simulink model "test_simmechanics_handling"  (Simulink 6.4)
settings: Solver=ode45  StartTime=0.0  StopTime=10  RelTol=1e-4  AbsTol=1e-4
InitFcn:
  | hFA = 0.2908;
  | hRA = 0.2909;
StopFcn:
  | subplot(3,1,1)
  | plot(time,velacc(:,8))
  | ylabel('lateral acceleration [m/s2]')
  | 
  | subplot(3,1,2)
  | plot(time,velacc(:,6))
  | ylabel('yaw velocity [deg/s]')
  | 
  | subplot(3,1,3)
  | plot(time,varinf1(:,3),time,varinf2(:,3),time,varinf3(:,3),time,varinf4(:,3))
  | xlabel('time [s]')
  | ylabel('vertical tyre force Fz [N]')
libraries: mblibv1 x31, Delft_Tyre_sm1glib x12
settings Model: Creator=luijtenmfj  LastModifiedBy=hofstadrhmtvd
settings DataIOCC: LimitDataPoints=off  SaveOutput=off  SignalLoggingName=sigsOut  OutputOption=SpecifiedOutputTimes  OutputTimes=[0:0.01:10]
settings DebuggingCC: SolverPrmCheckMsg=none  StrictBusMsg=ErrorLevel1
settings HardwareCC: TargetEndianess=LittleEndian  TargetHWDeviceType=MATLAB Host  ProdEqTarget=off
settings RTWCC: SystemTargetFile=rsim.tlc  TemplateMakefile=rsim_default_tmf  Description=Rapid Simulation Target  ProcessScript=rsim_make_rtw_hook
settings RSimTargetCC: TargetFcnLib=ansi_tfl_tmw.mat  GenFloatMathFcnCalls=ANSI_C  IsPILTarget=off  IncludeERTFirstTime=on
settings CustomProperty: DataType=string  Value=ANSI_C
settings SimMechanicsCC: VisDuringSimulation=on

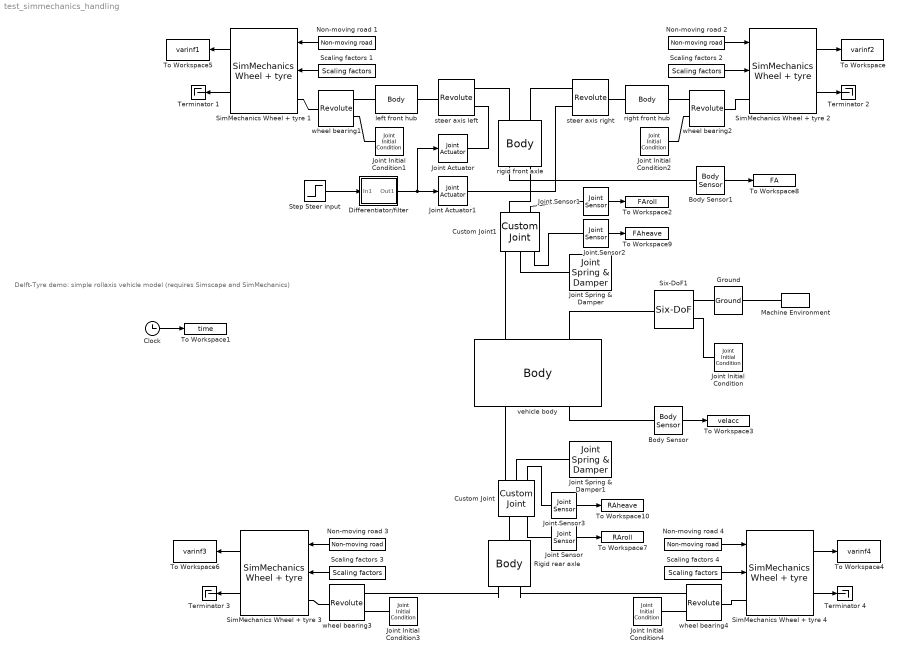
== system test_simmechanics_handling ==
  note: Delft-Tyre demo: simple rollaxis vehicle model
      | (requires Simscape and SimMechanics)
  Body Sensor : mblibv1/Sensors &  Actuators/Body Sensor  DialogController=MECH.DynMechDlgSource  SystemSampleTime=-1  PhysicalDomain=Mechanical  PortType=blob  Muxed=on  Pose=off  Angle=on  AngleUnits=deg  ArcVelocity=on  ArcVelocityUnits=deg/s  ArcAcceleration=off  ArcAccelerationUnits=deg/s^2  CoordPosition=off  CoordPositionUnits=m  Velocity=on  VelocityUnits=m/s  Acceleration=on  AccelerationUnits=m/s^2  Quaternion=on  QuaternionDT=off  QuaternionDDT=off  QuaternionUnits=off  OutputVector=[ 3 3 3 ]  ActiveIO=on  Width=9  DialogClass=MechanicalSensorBlock  ReferenceFrame=Local (Body CS)
  Body Sensor1 : mblibv1/Sensors &  Actuators/Body Sensor  DialogController=MECH.DynMechDlgSource  SystemSampleTime=-1  PhysicalDomain=Mechanical  PortType=blob  Muxed=on  Pose=off  Angle=on  AngleUnits=deg  ArcVelocity=off  ArcVelocityUnits=deg/s  ArcAcceleration=off  ArcAccelerationUnits=deg/s^2  CoordPosition=on  CoordPositionUnits=m  Velocity=off  VelocityUnits=m/s  Acceleration=off  AccelerationUnits=m/s^2  Quaternion=on  QuaternionDT=off  QuaternionDDT=off  QuaternionUnits=off  OutputVector=[ 3 ]  ActiveIO=on  Width=3  DialogClass=MechanicalSensorBlock  ReferenceFrame=Absolute (World)
  Clock : Clock
      settings: Decimation=10
  Custom Joint : mblibv1/Joints/Custom Joint  Orientation=down  DialogController=MECH.DynMechDlgSource  PhysicalDomain=mechanical  SubClassName=custom_joint  LeftPortType=blob  RightPortType=blob  LConnTagsString=__newl0|SA1|SA2  RConnTagsString=__newr0|SA1  NumSAPorts=3  CutJoint=off  MarkAsCut=off  Primitives=prismatic_revolute  PrimitiveProps=P1$WORLD$[0 0 1]$prismatic#R1$WORLD$[1 0 0]$revolute  DialogClass=JointBlock
  Custom Joint1 : mblibv1/Joints/Custom Joint  Orientation=up  DialogController=MECH.DynMechDlgSource  PhysicalDomain=mechanical  SubClassName=custom_joint  LeftPortType=blob  RightPortType=blob  LConnTagsString=__newl0|SA1|SA2  RConnTagsString=__newr0|SA1  NumSAPorts=3  CutJoint=off  MarkAsCut=off  Primitives=prismatic_revolute  PrimitiveProps=P1$WORLD$[0 0 1]$prismatic#R1$WORLD$[1 0 0]$revolute  DialogClass=JointBlock
  Differentiator/filter : Subsystem  mask{ts=0.05}
      mask prompts: ts "response_time"
      mask init:
      | c=(3*pi/ts)^2;
  Ground : mblibv1/Bodies/Ground  Orientation=left  DialogController=MECH.DynMechDlgSource  SystemSampleTime=-1  LeftPortType=env  RightPortType=workingframe  PhysicalDomain=Mechanical  DialogClass=GroundBlock  CoordPosition=[0 0 0]  CoordPositionUnits=m  StateVectorMgrId=-1  MachineId=[0 0]  ShowEnvPort=on
  Joint Actuator : mblibv1/Sensors &  Actuators/Joint Actuator  DialogController=MECH.DynMechDlgSource  SystemSampleTime=-1  PhysicalDomain=Mechanical  PortType=blob  ActuationStyle=Motion  AngleUnits=rad  ArcVelocityUnits=rad/s  ArcAccelerationUnits=rad/s^2  CoordPositionUnits=m  VelocityUnits=m/s  AccelerationUnits=m/s^2  ForceUnits=N  TorqueUnits=N-m  ActiveIO=on  Width=3  DialogClass=MechanicalActuatorBlock  Primitive=R1  ReferenceFrame=Absolute (INERTIAL)
  Joint Actuator1 : mblibv1/Sensors &  Actuators/Joint Actuator  DialogController=MECH.DynMechDlgSource  SystemSampleTime=-1  PhysicalDomain=Mechanical  PortType=blob  ActuationStyle=Motion  AngleUnits=rad  ArcVelocityUnits=rad/s  ArcAccelerationUnits=rad/s^2  CoordPositionUnits=m  VelocityUnits=m/s  AccelerationUnits=m/s^2  ForceUnits=N  TorqueUnits=N-m  ActiveIO=on  Width=3  DialogClass=MechanicalActuatorBlock  Primitive=R1  ReferenceFrame=Absolute (INERTIAL)
  Joint Initial Condition : mblibv1/Sensors &  Actuators/Joint Initial Condition  Orientation=left  DialogController=MECH.DynMechDlgSource  SystemSampleTime=-1  PhysicalDomain=Mechanical  DialogClass=InitialConditionBlock  InitialConditions=P1$true$0$m$rad$20$m/s$rad/s#P2$false$0$m$rad$0$m/s$rad/s#P3$false$-0.15$m$rad$0$m/s$rad/s#R1$false$0$m$rad$70$m/s$rad/s#R2$false$0$m$rad$0$m/s$rad/s#R3$false$0$m$rad$0$m/s$rad/s#S$false$0$m$rad$0$m/s$rad/s
  Joint Initial Condition1 : mblibv1/Sensors &  Actuators/Joint Initial Condition  Orientation=left  DialogController=MECH.DynMechDlgSource  SystemSampleTime=-1  PhysicalDomain=Mechanical  DialogClass=InitialConditionBlock  InitialConditions=P1$false$0$m$rad$20$m/s$rad/s#P2$false$0$m$rad$0$m/s$rad/s#P3$false$-0.15$m$rad$0$m/s$rad/s#R1$true$0$m$rad$66$m/s$rad/s#R2$false$0$m$rad$0$m/s$rad/s#R3$false$0$m$rad$0$m/s$rad/s#S$false$0$m$rad$0$m/s$rad/s
  Joint Initial Condition2 : mblibv1/Sensors &  Actuators/Joint Initial Condition  DialogController=MECH.DynMechDlgSource  SystemSampleTime=-1  PhysicalDomain=Mechanical  DialogClass=InitialConditionBlock  InitialConditions=P1$false$0$m$rad$20$m/s$rad/s#P2$false$0$m$rad$0$m/s$rad/s#P3$false$-0.15$m$rad$0$m/s$rad/s#R1$true$0$m$rad$66$m/s$rad/s#R2$false$0$m$rad$0$m/s$rad/s#R3$false$0$m$rad$0$m/s$rad/s#S$false$0$m$rad$0$m/s$rad/s
  Joint Initial Condition3 : mblibv1/Sensors &  Actuators/Joint Initial Condition  Orientation=left  DialogController=MECH.DynMechDlgSource  SystemSampleTime=-1  PhysicalDomain=Mechanical  DialogClass=InitialConditionBlock  InitialConditions=P1$false$0$m$rad$20$m/s$rad/s#P2$false$0$m$rad$0$m/s$rad/s#P3$false$-0.15$m$rad$0$m/s$rad/s#R1$true$0$m$rad$66$m/s$rad/s#R2$false$0$m$rad$0$m/s$rad/s#R3$false$0$m$rad$0$m/s$rad/s#S$false$0$m$rad$0$m/s$rad/s
  Joint Initial Condition4 : mblibv1/Sensors &  Actuators/Joint Initial Condition  DialogController=MECH.DynMechDlgSource  SystemSampleTime=-1  PhysicalDomain=Mechanical  DialogClass=InitialConditionBlock  InitialConditions=P1$false$0$m$rad$20$m/s$rad/s#P2$false$0$m$rad$0$m/s$rad/s#P3$false$-0.15$m$rad$0$m/s$rad/s#R1$true$0$m$rad$66$m/s$rad/s#R2$false$0$m$rad$0$m/s$rad/s#R3$false$0$m$rad$0$m/s$rad/s#S$false$0$m$rad$0$m/s$rad/s
  Joint Sensor : mblibv1/Sensors &  Actuators/Joint Sensor  DialogController=MECH.DynMechDlgSource  SystemSampleTime=-1  PhysicalDomain=Mechanical  PortType=blob  Muxed=on  Pose=off  Angle=on  AngleUnits=deg  ArcVelocity=on  ArcVelocityUnits=rad/s  ArcAcceleration=off  ArcAccelerationUnits=deg/s^2  CoordPosition=on  CoordPositionUnits=m  Velocity=off  VelocityUnits=m/s  Acceleration=off  AccelerationUnits=m/s^2  Quaternion=on  QuaternionDT=off  QuaternionDDT=off  QuaternionUnits=off  OutputVector=[ 1 1 3 ]  ActiveIO=on  Width=5  DialogClass=MechanicalSensorBlock  Primitive=R1  Force=off  ForceUnits=N  Torque=off  TorqueUnits=N-m  ReferenceFrame=Absolute (INERTIAL)  ReactionSensedSide=Base  ReactionReferenceFrame=Absolute (World)  ReactionForce=on  ReactionForceUnits=N  ReactionMoment=off  ReactionMomentUnits=N-m
  Joint Sensor1 : mblibv1/Sensors &  Actuators/Joint Sensor  DialogController=MECH.DynMechDlgSource  SystemSampleTime=-1  PhysicalDomain=Mechanical  PortType=blob  Muxed=on  Pose=off  Angle=on  AngleUnits=deg  ArcVelocity=on  ArcVelocityUnits=rad/s  ArcAcceleration=off  ArcAccelerationUnits=deg/s^2  CoordPosition=on  CoordPositionUnits=m  Velocity=off  VelocityUnits=m/s  Acceleration=off  AccelerationUnits=m/s^2  Quaternion=on  QuaternionDT=off  QuaternionDDT=off  QuaternionUnits=off  OutputVector=[ 1 1 3 ]  ActiveIO=on  Width=5  DialogClass=MechanicalSensorBlock  Primitive=R1  Force=off  ForceUnits=N  Torque=off  TorqueUnits=N-m  ReferenceFrame=Absolute (INERTIAL)  ReactionSensedSide=Base  ReactionReferenceFrame=Absolute (World)  ReactionForce=on  ReactionForceUnits=N  ReactionMoment=off  ReactionMomentUnits=N-m
  Joint Sensor2 : mblibv1/Sensors &  Actuators/Joint Sensor  DialogController=MECH.DynMechDlgSource  SystemSampleTime=-1  PhysicalDomain=Mechanical  PortType=blob  Muxed=on  Pose=off  Angle=on  AngleUnits=deg  ArcVelocity=on  ArcVelocityUnits=deg/s  ArcAcceleration=off  ArcAccelerationUnits=deg/s^2  CoordPosition=on  CoordPositionUnits=m  Velocity=on  VelocityUnits=m/s  Acceleration=off  AccelerationUnits=m/s^2  Quaternion=on  QuaternionDT=off  QuaternionDDT=off  QuaternionUnits=off  OutputVector=[ 1 1 3 ]  ActiveIO=on  Width=5  DialogClass=MechanicalSensorBlock  Primitive=P1  Force=off  ForceUnits=N  Torque=off  TorqueUnits=N-m  ReferenceFrame=Absolute (INERTIAL)  ReactionSensedSide=Base  ReactionReferenceFrame=Absolute (World)  ReactionForce=on  ReactionForceUnits=N  ReactionMoment=off  ReactionMomentUnits=N-m
  Joint Sensor3 : mblibv1/Sensors &  Actuators/Joint Sensor  DialogController=MECH.DynMechDlgSource  SystemSampleTime=-1  PhysicalDomain=Mechanical  PortType=blob  Muxed=on  Pose=off  Angle=on  AngleUnits=deg  ArcVelocity=on  ArcVelocityUnits=deg/s  ArcAcceleration=off  ArcAccelerationUnits=deg/s^2  CoordPosition=on  CoordPositionUnits=m  Velocity=on  VelocityUnits=m/s  Acceleration=off  AccelerationUnits=m/s^2  Quaternion=on  QuaternionDT=off  QuaternionDDT=off  QuaternionUnits=off  OutputVector=[ 1 1 3 ]  ActiveIO=on  Width=5  DialogClass=MechanicalSensorBlock  Primitive=P1  Force=off  ForceUnits=N  Torque=off  TorqueUnits=N-m  ReferenceFrame=Absolute (INERTIAL)  ReactionSensedSide=Base  ReactionReferenceFrame=Absolute (World)  ReactionForce=on  ReactionForceUnits=N  ReactionMoment=off  ReactionMomentUnits=N-m
  Joint Spring & Damper : mblibv1/Force  Elements/Joint Spring & Damper  DialogController=MECH.DynMechDlgSource  SystemSampleTime=-1  DialogClass=JointSpringDamper  JFEParameters=P1$true$40000$3500$-.20$m$m/s$N$rad$rad/s$N-m#P2$false$0$0$0$m$m/s$N$rad$rad/s$N-m#P3$false$0$0$0$m$m/s$N$rad$rad/s$N-m#R1$true$66000$2050$0$m$m/s$N$rad$rad/s$N-m#R2$false$0$0$0$m$m/s$N$rad$rad/s$N-m#R3$false$0$0$0$m$m/s$N$rad$rad/s$N-m#S$false$0$0$0$m$m/s$N$rad$rad/s$N-m
  Joint Spring & Damper1 : mblibv1/Force  Elements/Joint Spring & Damper  DialogController=MECH.DynMechDlgSource  SystemSampleTime=-1  DialogClass=JointSpringDamper  JFEParameters=P1$true$50000$3500$-0.16$m$m/s$N$rad$rad/s$N-m#P2$false$0$0$0$m$m/s$N$rad$rad/s$N-m#P3$false$0$0$0$m$m/s$N$rad$rad/s$N-m#R1$true$27500$2050$0$m$m/s$N$rad$rad/s$N-m#R2$false$0$0$0$m$m/s$N$rad$rad/s$N-m#R3$false$0$0$0$m$m/s$N$rad$rad/s$N-m#S$false$0$0$0$m$m/s$N$rad$rad/s$N-m
  Machine Environment : mblibv1/Bodies/Machine Environment  Tag=Factory ground  Orientation=left  DialogController=MECH.DialogSource  SystemSampleTime=-1  PortType=env  PhysicalDomain=Mechanical  DialogTemplateClass=MECH.MachineEnvironment  SyncWhenCopied=off  Gravity=[0 0 -10]  GravityUnits=m/s^2  GravityAsSignal=off  Dimensionality=Auto-detect  AnalysisType=Forward dynamics  LinearAssemblyTolerance=1e-3  LinearAssemblyToleranceUnits=m  AngularAssemblyTolerance=1e-3  AngularAssemblyToleranceUnits=rad  ConstraintSolverType=Stabilizing  ConstraintRelTolerance=1e-4  ConstraintAbsTolerance=1e-4  UseRobustSingularityHandling=off  StatePerturbationType=Fixed  PerturbationSize=1e-5  VisualizeMachine=on
  Non-moving road 1 : Delft_Tyre_sm1glib/SimMechanics 1G/Non-moving road  Orientation=left  SystemSampleTime=-1  dummy=off
  Non-moving road 2 : Delft_Tyre_sm1glib/SimMechanics 1G/Non-moving road  SystemSampleTime=-1  dummy=off
  Non-moving road 3 : Delft_Tyre_sm1glib/SimMechanics 1G/Non-moving road  Orientation=left  SystemSampleTime=-1  dummy=off
  Non-moving road 4 : Delft_Tyre_sm1glib/SimMechanics 1G/Non-moving road  SystemSampleTime=-1  dummy=off
  Rigid rear axle : mblibv1/Bodies/Body  Orientation=down  DialogController=MECH.DynMechDlgSource  PhysicalDomain=mechanical  SubClassName=Unknown  LeftPortType=workingframe  RightPortType=workingframe  LConnTagsString=CS1  RConnTagsString=CS2|CS3  DialogClass=MechanicalBodyBlock  Mass=90  MassUnits=kg  InertiaUnits=kg*m^2  Inertia=eye(3)  Shape=Cylinder  ShapeDims=[1 1]  ShapeUnits=m  ShapeUse=false  Density=1  DensityUnits=kg/m^3  DensityUse=false  CG=Left$CG$[-3 0 hRA]$WORLD$WORLD$m$[0 0 0]$Euler X-Y-Z$deg$WORLD$false$none  WorkingFrames=Left$CS1$[-3 0 0.05]$WORLD$WORLD$m$[0 0 0]$Euler X-Y-Z$deg$WORLD$true$none#Right$CS2$[-3 0.80 hRA]$WORLD$WORLD$m$[0 0 0]$Euler X-Y-Z$deg$WORLD$true$none#Right$CS3$[-3 -0.80 hRA]$WORLD$WORLD$m$[0 0 0]$Euler X-Y-Z$deg$WORLD$true$none
  Scaling factors 1 : Delft_Tyre_sm1glib/SimMechanics 1G/Scaling factors  Orientation=left  SystemSampleTime=-1  LMUX=1  LKX=1  LMUY=1  LKY=1  LKYC=1  LTR=1  LKZC=1
  Scaling factors 2 : Delft_Tyre_sm1glib/SimMechanics 1G/Scaling factors  SystemSampleTime=-1  LMUX=1  LKX=1  LMUY=1  LKY=1  LKYC=1  LTR=1  LKZC=1
  Scaling factors 3 : Delft_Tyre_sm1glib/SimMechanics 1G/Scaling factors  Orientation=left  SystemSampleTime=-1  LMUX=1  LKX=1  LMUY=1  LKY=1  LKYC=1  LTR=1  LKZC=1
  Scaling factors 4 : Delft_Tyre_sm1glib/SimMechanics 1G/Scaling factors  SystemSampleTime=-1  LMUX=1  LKX=1  LMUY=1  LKY=1  LKYC=1  LTR=1  LKZC=1
  SimMechanics Wheel + tyre 1 : Delft_Tyre_sm1glib/SimMechanics 1G/SimMechanics Wheel + tyre  Tag=SimMechanics Wheel + tyre  Orientation=left  SystemSampleTime=-1  idtyre=1  inertia=[10 1 2]  tpfname='TNO_car205_60R15.tir'  rdfname='TNO_FlatRoad.rdf'  side_mode=(1xxx) left  cnt_mode=(x1xx) smooth road  dyn_mode=(xx0x) steady-state  mf_mode=(xxx4) combined  use_mode=1e8  disp_debug=off
  SimMechanics Wheel + tyre 2 : Delft_Tyre_sm1glib/SimMechanics 1G/SimMechanics Wheel + tyre  Tag=SimMechanics Wheel + tyre  SystemSampleTime=-1  idtyre=2  inertia=[10 1 2]  tpfname='TNO_car205_60R15.tir'  rdfname='TNO_FlatRoad.rdf'  side_mode=(2xxx) right  cnt_mode=(x1xx) smooth road  dyn_mode=(xx0x) steady-state  mf_mode=(xxx4) combined  use_mode=1e8  disp_debug=off
  SimMechanics Wheel + tyre 3 : Delft_Tyre_sm1glib/SimMechanics 1G/SimMechanics Wheel + tyre  Tag=SimMechanics Wheel + tyre  Orientation=left  SystemSampleTime=-1  idtyre=3  inertia=[10 1 2]  tpfname='TNO_car205_60R15.tir'  rdfname='TNO_FlatRoad.rdf'  side_mode=(1xxx) left  cnt_mode=(x1xx) smooth road  dyn_mode=(xx0x) steady-state  mf_mode=(xxx4) combined  use_mode=1e8  disp_debug=off
  SimMechanics Wheel + tyre 4 : Delft_Tyre_sm1glib/SimMechanics 1G/SimMechanics Wheel + tyre  Tag=SimMechanics Wheel + tyre  SystemSampleTime=-1  idtyre=4  inertia=[10 1 2]  tpfname='TNO_car205_60R15.tir'  rdfname='TNO_FlatRoad.rdf'  side_mode=(2xxx) right  cnt_mode=(x1xx) smooth road  dyn_mode=(xx0x) steady-state  mf_mode=(xxx4) combined  use_mode=1e8  disp_debug=off
  Six-DoF1 : mblibv1/Joints/Six-DoF  Orientation=left  DialogController=MECH.DynMechDlgSource  PhysicalDomain=mechanical  SubClassName=Unknown  LeftPortType=blob  RightPortType=blob  LConnTagsString=__newl0|SA1  RConnTagsString=__newr0  NumSAPorts=1  CutJoint=off  MarkAsCut=off  Primitives=prismatic_prismatic_prismatic_spherical  PrimitiveProps=P1$WORLD$[1 0 0]$prismatic#P2$WORLD$[0 1 0]$prismatic#P3$WORLD$[0 0 1]$prismatic#S$WORLD$[0 0 0]$spherical  DialogClass=JointBlock
  Step Steer input : Step  Time=3  After=10*pi/180  SampleTime=0
  Terminator {1..4} (4 alike) : Terminator
  To Workspace : ToWorkspace  VariableName=varinf2  SampleTime=-1  SaveFormat=Array
  To Workspace1 : ToWorkspace  VariableName=time  SampleTime=-1  SaveFormat=Array
  To Workspace10 : ToWorkspace  VariableName=RAheave  SampleTime=-1  SaveFormat=Array
  To Workspace2 : ToWorkspace  VariableName=FAroll  SampleTime=-1  SaveFormat=Array
  To Workspace3 : ToWorkspace  VariableName=velacc  SampleTime=-1  SaveFormat=Array
  To Workspace4 : ToWorkspace  VariableName=varinf4  SampleTime=-1  SaveFormat=Array
  To Workspace5 : ToWorkspace  VariableName=varinf1  SampleTime=-1  SaveFormat=Array
  To Workspace6 : ToWorkspace  VariableName=varinf3  SampleTime=-1  SaveFormat=Array
  To Workspace7 : ToWorkspace  VariableName=RAroll  SampleTime=-1  SaveFormat=Array
  To Workspace8 : ToWorkspace  VariableName=FA  SampleTime=-1  SaveFormat=Array
  To Workspace9 : ToWorkspace  VariableName=FAheave  SampleTime=-1  SaveFormat=Array
  left front hub : mblibv1/Bodies/Body  Orientation=left  DialogController=MECH.DynMechDlgSource  PhysicalDomain=mechanical  SubClassName=Unknown  LeftPortType=workingframe  RightPortType=workingframe  LConnTagsString=CS1  RConnTagsString=CS2  DialogClass=MechanicalBodyBlock  Mass=0  MassUnits=kg  InertiaUnits=kg*m^2  Inertia=zeros(3)  Shape=Cylinder  ShapeDims=[1 1]  ShapeUnits=m  ShapeUse=false  Density=1  DensityUnits=kg/m^3  DensityUse=false  CG=Left$CG$[0 0.80 hFA]$WORLD$WORLD$m$[0 0 0]$Euler X-Y-Z$deg$WORLD$false$none  WorkingFrames=Left$CS1$[0 0 0]$CG$CG$m$[0 0 0]$Euler X-Y-Z$deg$WORLD$true$none#Right$CS2$[0 0 0]$CG$CG$m$[0 0 0]$Euler X-Y-Z$deg$WORLD$true$none
  right front hub : mblibv1/Bodies/Body  DialogController=MECH.DynMechDlgSource  PhysicalDomain=mechanical  SubClassName=Unknown  LeftPortType=workingframe  RightPortType=workingframe  LConnTagsString=CS1  RConnTagsString=CS2  DialogClass=MechanicalBodyBlock  Mass=0  MassUnits=kg  InertiaUnits=kg*m^2  Inertia=zeros(3)  Shape=Cylinder  ShapeDims=[1 1]  ShapeUnits=m  ShapeUse=false  Density=1  DensityUnits=kg/m^3  DensityUse=false  CG=Left$CG$[0 -0.80 hFA]$WORLD$WORLD$m$[0 0 0]$Euler X-Y-Z$deg$WORLD$false$none  WorkingFrames=Left$CS1$[0 0 0]$CG$CG$m$[0 0 0]$Euler X-Y-Z$deg$WORLD$true$none#Right$CS2$[0 0 0]$CG$CG$m$[0 0 0]$Euler X-Y-Z$deg$WORLD$true$none
  rigid front axle : mblibv1/Bodies/Body  Orientation=up  DialogController=MECH.DynMechDlgSource  PhysicalDomain=mechanical  SubClassName=Unknown  LeftPortType=workingframe  RightPortType=workingframe  LConnTagsString=CG|CS1  RConnTagsString=CS2|CS3  DialogClass=MechanicalBodyBlock  Mass=95  MassUnits=kg  InertiaUnits=kg*m^2  Inertia=eye(3)  Shape=Cylinder  ShapeDims=[1 1]  ShapeUnits=m  ShapeUse=false  Density=1  DensityUnits=kg/m^3  DensityUse=false  CG=Left$CG$[0 0 hFA]$WORLD$WORLD$m$[0 0 0]$Euler X-Y-Z$deg$WORLD$true$none  WorkingFrames=Left$CS1$[0 0 -hFA]$CG$CG$m$[0 0 0]$Euler X-Y-Z$deg$WORLD$true$none#Right$CS2$[0 0.80 hFA]$WORLD$WORLD$m$[0 0 0]$Euler X-Y-Z$deg$WORLD$true$none#Right$CS3$[0 -0.80 hFA]$WORLD$WORLD$m$[0 0 0]$Euler X-Y-Z$deg$WORLD$true$none
  steer axis left : mblibv1/Joints/Revolute  Orientation=left  DialogController=MECH.DynMechDlgSource  PhysicalDomain=mechanical  SubClassName=Unknown  LeftPortType=blob  RightPortType=blob  LConnTagsString=__newl0|SA1  RConnTagsString=__newr0  NumSAPorts=1  CutJoint=off  MarkAsCut=off  Primitives=revolute  PrimitiveProps=R1$WORLD$[0 0 1]$revolute  DialogClass=JointBlock
  steer axis right : mblibv1/Joints/Revolute  DialogController=MECH.DynMechDlgSource  PhysicalDomain=mechanical  SubClassName=Unknown  LeftPortType=blob  RightPortType=blob  LConnTagsString=__newl0|SA1  RConnTagsString=__newr0  NumSAPorts=1  CutJoint=off  MarkAsCut=off  Primitives=revolute  PrimitiveProps=R1$WORLD$[0 0 1]$revolute  DialogClass=JointBlock
  vehicle body : mblibv1/Bodies/Body  Orientation=down  DialogController=MECH.DynMechDlgSource  PhysicalDomain=mechanical  SubClassName=Unknown  LeftPortType=workingframe  RightPortType=workingframe  LConnTagsString=CS1|CG  RConnTagsString=CS2|CS7  DialogClass=MechanicalBodyBlock  Mass=1600  MassUnits=kg  InertiaUnits=kg*m^2  Inertia=[600 0 0; 0 3000 0 ; 0 0 3200]  Shape=Cylinder  ShapeDims=[1 1]  ShapeUnits=m  ShapeUse=false  Density=1  DensityUnits=kg/m^3  DensityUse=false  CG=Left$CG$[-1.5 0 0.55]$WORLD$WORLD$m$[0 0 0]$Euler X-Y-Z$deg$WORLD$true  WorkingFrames=Left$CS1$[0 0 0.10]$WORLD$WORLD$m$[0 0 0]$Euler X-Y-Z$deg$WORLD$true#Right$CS2$[-3 0 0.10]$WORLD$WORLD$m$[0 0 0]$Euler X-Y-Z$deg$WORLD$true#Right$CS7$[0 0 0]$CG$CG$m$[0 0 0]$Euler X-Y-Z$deg$WORLD$true#Right$CS3$[0 0.5 0.5]$WORLD$WORLD$m$[0 0 0]$Euler X-Y-Z$deg$WORLD$false#Right$CS4$[0 -0.5 0.5]$WORLD$WORLD$m$[0 0 0]$Euler X-Y-Z$deg$WORLD$false#Right$CS5$[-3 -0.5 0.5]$WORLD$WORLD$m$[0 0 0]$Euler X-Y-Z$deg$WORLD$false#Right$CS6$[-3 0.5 0.5]$WORLD$WORLD$m$[0 0 0]$Euler X-Y-Z$deg$WORLD$false
  wheel bearing1 : mblibv1/Joints/Revolute  Orientation=left  DialogController=MECH.DynMechDlgSource  PhysicalDomain=mechanical  SubClassName=Unknown  LeftPortType=blob  RightPortType=blob  LConnTagsString=__newl0|SA1  RConnTagsString=__newr0  NumSAPorts=1  CutJoint=off  MarkAsCut=off  Primitives=revolute  PrimitiveProps=R1$Base$[0 1 0]$revolute  DialogClass=JointBlock
  wheel bearing2 : mblibv1/Joints/Revolute  DialogController=MECH.DynMechDlgSource  PhysicalDomain=mechanical  SubClassName=Unknown  LeftPortType=blob  RightPortType=blob  LConnTagsString=__newl0|SA1  RConnTagsString=__newr0  NumSAPorts=1  CutJoint=off  MarkAsCut=off  Primitives=revolute  PrimitiveProps=R1$Base$[0 1 0]$revolute  DialogClass=JointBlock
  wheel bearing3 : mblibv1/Joints/Revolute  Orientation=left  DialogController=MECH.DynMechDlgSource  PhysicalDomain=mechanical  SubClassName=Unknown  LeftPortType=blob  RightPortType=blob  LConnTagsString=__newl0|SA1  RConnTagsString=__newr0  NumSAPorts=1  CutJoint=off  MarkAsCut=off  Primitives=revolute  PrimitiveProps=R1$Base$[0 1 0]$revolute  DialogClass=JointBlock
  wheel bearing4 : mblibv1/Joints/Revolute  DialogController=MECH.DynMechDlgSource  PhysicalDomain=mechanical  SubClassName=Unknown  LeftPortType=blob  RightPortType=blob  LConnTagsString=__newl0|SA1  RConnTagsString=__newr0  NumSAPorts=1  CutJoint=off  MarkAsCut=off  Primitives=revolute  PrimitiveProps=R1$Base$[0 1 0]$revolute  DialogClass=JointBlock
  wires:
  SimMechanics Wheel + tyre 2/1 -> To Workspace/1
  SimMechanics Wheel + tyre 1/1 -> To Workspace5/1
  SimMechanics Wheel + tyre 3/1 -> To Workspace6/1
  Differentiator/filter/1(Out1) -> Joint Actuator/1, Joint Actuator1/1
  Clock/1 -> To Workspace1/1
  Body Sensor/1 -> To Workspace3/1
  Step Steer input/1 -> Differentiator/filter/1(In1)
  Joint Sensor1/1 -> To Workspace2/1
  Joint Sensor/1 -> To Workspace7/1
  Body Sensor1/1 -> To Workspace8/1
  Joint Sensor2/1 -> To Workspace9/1
  Joint Sensor3/1 -> To Workspace10/1
  Non-moving road 1/1 -> SimMechanics Wheel + tyre 1/1
  Scaling factors 1/1 -> SimMechanics Wheel + tyre 1/2
  SimMechanics Wheel + tyre 1/2 -> Terminator 1/1
  SimMechanics Wheel + tyre 2/2 -> Terminator 2/1
  Non-moving road 2/1 -> SimMechanics Wheel + tyre 2/1
  Scaling factors 2/1 -> SimMechanics Wheel + tyre 2/2
  Non-moving road 3/1 -> SimMechanics Wheel + tyre 3/1
  Scaling factors 3/1 -> SimMechanics Wheel + tyre 3/2
  SimMechanics Wheel + tyre 3/2 -> Terminator 3/1
  Non-moving road 4/1 -> SimMechanics Wheel + tyre 4/1
  Scaling factors 4/1 -> SimMechanics Wheel + tyre 4/2
  SimMechanics Wheel + tyre 4/1 -> To Workspace4/1
  SimMechanics Wheel + tyre 4/2 -> Terminator 4/1
  connections:
  wheel bearing2/RConn1 -- SimMechanics Wheel + tyre 2/LConn1
  wheel bearing1/RConn1 -- SimMechanics Wheel + tyre 1/LConn1
  Rigid rear axle/RConn2 -- wheel bearing4/LConn1
  Rigid rear axle/RConn1 -- wheel bearing3/LConn1
  wheel bearing3/RConn1 -- SimMechanics Wheel + tyre 3/LConn1
  Custom Joint/RConn1 -- Rigid rear axle/LConn1
  vehicle body/RConn1 -- Custom Joint/LConn1
  Ground/RConn1 -- Six-DoF1/LConn1
  Joint Initial Condition/RConn1 -- Six-DoF1/LConn2
  Custom Joint1/RConn1 -- rigid front axle/LConn2
  wheel bearing4/RConn1 -- SimMechanics Wheel + tyre 4/LConn1
  right front hub/RConn1 -- wheel bearing2/LConn1
  left front hub/RConn1 -- wheel bearing1/LConn1
  steer axis right/RConn1 -- right front hub/LConn1
  rigid front axle/RConn2 -- steer axis right/LConn1
  steer axis left/RConn1 -- left front hub/LConn1
  rigid front axle/RConn1 -- steer axis left/LConn1
  Joint Actuator/RConn1 -- steer axis left/LConn2
  Joint Actuator1/RConn1 -- steer axis right/LConn2
  Custom Joint1/LConn2 -- Joint Spring & Damper/LConn1
  vehicle body/LConn1 -- Custom Joint1/LConn1
  vehicle body/LConn2 -- Six-DoF1/RConn1
  vehicle body/RConn2 -- Body Sensor/LConn1
  Joint Spring & Damper1/LConn1 -- Custom Joint/LConn2
  Joint Sensor/LConn1 -- Custom Joint/RConn2
  Joint Sensor1/LConn1 -- Custom Joint1/RConn2
  Body Sensor1/LConn1 -- rigid front axle/LConn1
  Joint Sensor2/LConn1 -- Custom Joint1/LConn3
  Custom Joint/LConn3 -- Joint Sensor3/LConn1
  Machine Environment/RConn1 -- Ground/LConn1
  Joint Initial Condition1/RConn1 -- wheel bearing1/LConn2
  Joint Initial Condition2/RConn1 -- wheel bearing2/LConn2
  Joint Initial Condition3/RConn1 -- wheel bearing3/LConn2
  Joint Initial Condition4/RConn1 -- wheel bearing4/LConn2

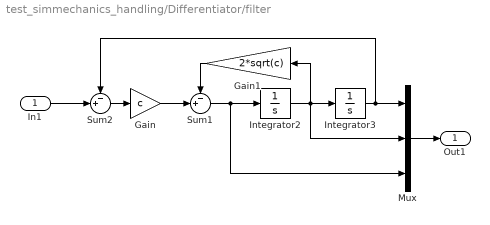
== system test_simmechanics_handling/Differentiator/filter ==
  In1 : Inport
  Gain : Gain  Gain=c  SaturateOnIntegerOverflow=on
  Gain1 : Gain  Orientation=left  Gain=2*sqrt(c)  SaturateOnIntegerOverflow=on
  Integrator2 : Integrator
  Integrator3 : Integrator
  Mux : Mux  Inputs=3
  Sum1 : Sum  Inputs=-+|  SaturateOnIntegerOverflow=on
  Sum2 : Sum  Inputs=-+|  SaturateOnIntegerOverflow=on
  Out1 : Outport
  wires:
  Integrator2/1 -> Integrator3/1, Mux/2, Gain1/1
  Integrator3/1 -> Mux/1, Sum2/1
  Mux/1 -> Out1/1
  Sum1/1 -> Mux/3, Integrator2/1
  Sum2/1 -> Gain/1
  In1/1 -> Sum2/2
  Gain1/1 -> Sum1/1
  Gain/1 -> Sum1/2
